simulink model "CircuitoOdeSIMULINK"  (R2024b)
settings: Solver=VariableStepAuto  StartTime=0.0  StopTime=.002  MaxStep=.0000001  RelTol=1e-3
settings Model: Creator=Charles
settings SolverCC: AlgebraicLoopSolver=TrustRegion
settings DataIOCC: ReturnWorkspaceOutputs=off
settings DebuggingCC: UnconnectedInputMsg=warning  UnconnectedOutputMsg=warning  UnconnectedLineMsg=warning  ArithmeticOperatorsInVariantConditions=warning
settings ModelReferenceCC: EnableRefExpFcnMdlSchedulingChecks=on
settings SFSimCC: SimUseLocalCustomCode=off  CustomCodeUndefinedFunction=UseInterfaceOnly
settings RTWCC: RTWUseLocalCustomCode=off  GPUComputeCapability=3.5

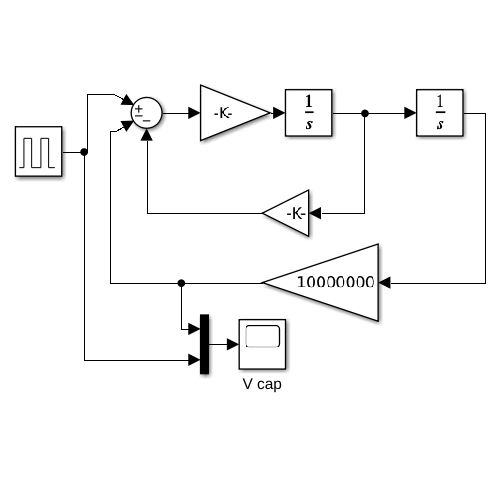
[thumbnail: Simulink's stored preview of the top-level diagram]
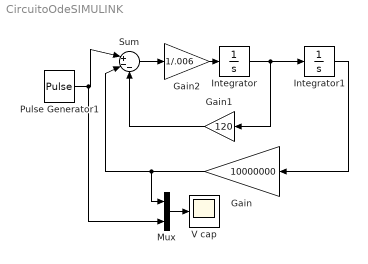
== system CircuitoOdeSIMULINK ==
  Gain : Gain  Gain=10000000
  Gain1 : Gain  Gain=120
  Gain2 : Gain  Gain=1/.006
  Integrator : Integrator
  Integrator1 : Integrator
  Mux : Mux  Inputs=2
  Pulse Generator1 : DiscretePulseGenerator  PulseType=Time based  Amplitude=5  Period=.002  PulseWidth=50
  Sum : Sum  Inputs=|+--
  "V cap " : Scope
  wires:
  Gain/1 -> Mux/1, Sum/2
  Gain1/1 -> Sum/3
  Sum/1 -> Gain2/1
  Gain2/1 -> Integrator/1
  Integrator/1 -> Gain1/1, Integrator1/1
  Integrator1/1 -> Gain/1
  Pulse Generator1/1 -> Mux/2, Sum/1
  Mux/1 -> "V cap "/1
